simulink model "audio_sine_wave"  (R2023a)
settings: Solver=FixedStepAuto  StartTime=0.0  StopTime=10.0  RelTol=1e-3
undefined symbols (not defined in the file): Data_Display, untitled2
libraries: androidsensorlib x1, androidaudiovideolib x1, androiduilib x1
settings Model: Creator=ragha  LastModifiedBy=ragha
settings OptimizationCC: EnhancedBackFolding=on  PassReuseOutputArgsAs=Individual arguments  ZeroExternalMemoryAtStartup=off  ZeroInternalMemoryAtStartup=off  MaxStackSize=64  OptimizeBlockOrder=speed  DifferentSizesBufferReuse=on  OptimizationCustomize=off  EfficientTunableParamExpr=on
settings DebuggingCC: ParameterTunabilityLossMsg=error
settings HardwareCC: ProdBitPerPointer=32  ProdBitPerSizeT=32  ProdBitPerPtrDiffT=32  ProdLargestAtomicInteger=Long  ProdLargestAtomicFloat=Double  ProdWordSize=32  ProdHWDeviceType=ARM Compatible->ARM Cortex
settings SFSimCC: MATLABDynamicMemAlloc=off
settings RTWCC: Description=Embedded Coder  SystemTargetFile=ert.tlc  HardwareBoard=Android Device  TLCOptions="-aInlineSetEventsForThisBaseRateFcn=TLC_FALSE -aSuppressMultiTaskScheduler=TLC_FALSE  -aRateBasedStepFcn=0"  TemplateMakefile=ert_default_tmf  RTWVerbose=off  Toolchain=Android SDK/NDK Tools
settings CodeAppCC: ForceParamTrailComments=on  IgnoreCustomStorageClasses=off  OperatorAnnotations=on  SimulinkDataObjDesc=on  SFDataObjDesc=on  InsertBlockDesc=on

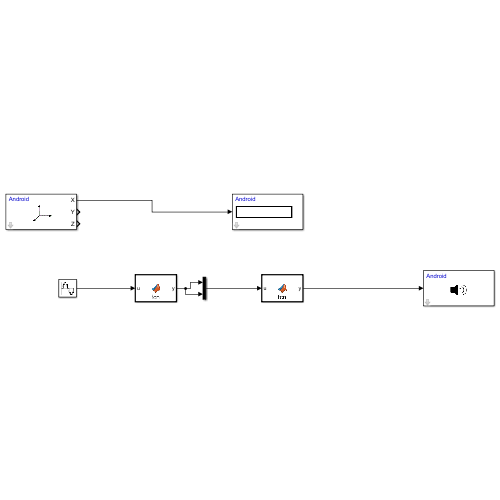
[thumbnail: Simulink's stored preview of the top-level diagram]
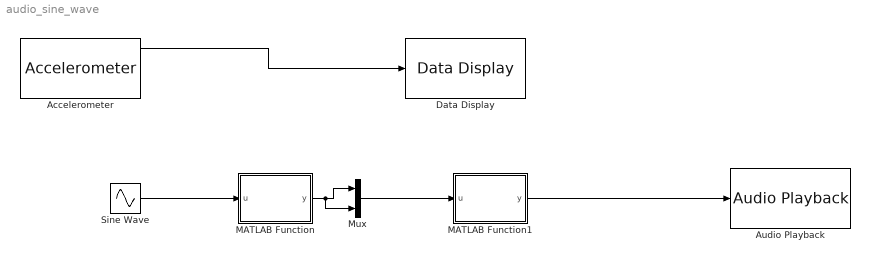
== system audio_sine_wave ==
  Accelerometer : androidsensorlib/Accelerometer  OutputVector=off  SampleTime=0.1  BlockPlatform=Android
  Audio Playback : androidaudiovideolib/Audio Playback  SampleFreq=44100  AudioSamplingFreq=44100  SampleTime=0.1  DeviceStr=0  QueueDuration=0  BlockPlatform=Android
  Data Display : androiduilib/Data Display  DataDisplayId=untitled2/Data_Display  Format=Float  Precision=6  SimulateUsing=Code generation  blockPlatform=Android
  MATLAB Function : MATLAB Function  TreatAsAtomicUnit=on
  MATLAB Function1 : MATLAB Function  TreatAsAtomicUnit=on
  Mux : Mux  Inputs=2
  Sine Wave : Sin  Amplitude=10000/2  Frequency=2.*pi.*10000  SampleTime=1/44100  VectorParams1D=off
  wires:
  Sine Wave/1 -> MATLAB Function/1(u)
  Accelerometer/1 -> Data Display/1
  MATLAB Function/1(y) -> Mux/2, Mux/1
  Mux/1 -> MATLAB Function1/1(u)
  MATLAB Function1/1(y) -> Audio Playback/1

== matlab function audio_sine_wave/MATLAB Function ==
  data: u input; y output
function y = fcn(u)
    u = int16(u);
y = u;

== matlab function audio_sine_wave/MATLAB Function1 ==
  data: u input; y output
function y = fcn(u)
    u = u';
y = u;
